simulink model "practica3_PT"  (R2015a)
settings: Solver=ode4  StartTime=0.0  StopTime=1  FixedStep=.005  RelTol=1e-3
settings Model: Creator=Sala6  LastModifiedBy=Jesus

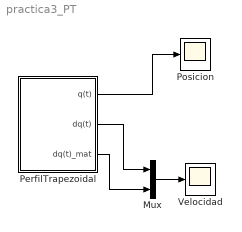
== system practica3_PT ==
  Mux : Mux  Inputs=2
  PerfilTrapezoidal : Subsystem  mask{tf=1, V=60, q0=0, qf=40}
      mask prompts: tf "Tiempo final"; V "Velocidad del perfil"; q0 "Posicion inicial"; qf "Posicion final"
      mask init:
      | % tiempo de mezcla
      | tb=(q0-qf+V*tf)/V
      | a=V/tb
  Posicion : Scope
  Velocidad : Scope
  wires:
  Mux/1 -> Velocidad/1
  PerfilTrapezoidal/2(dq(t)) -> Mux/1
  PerfilTrapezoidal/3(dq(t)_mat) -> Mux/2
  PerfilTrapezoidal/1("q(t) ") -> Posicion/1

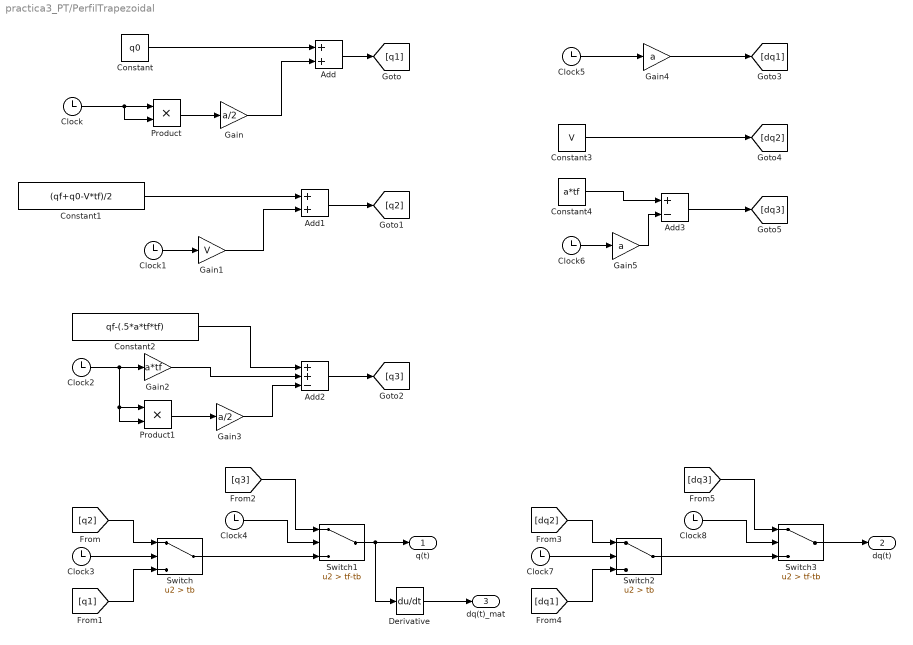
== system practica3_PT/PerfilTrapezoidal ==
  Add : Sum
  Add1 : Sum
  Add2 : Sum  Inputs=++-
  Add3 : Sum  Inputs=+-
  Clock{,1..8} (9 alike) : Clock
  Constant : Constant  Value=q0
  Constant1 : Constant  Value=(qf+q0-V*tf)/2
  Constant2 : Constant  Value=qf-(.5*a*tf*tf)
  Constant3 : Constant  Value=V
  Constant4 : Constant  Value=a*tf
  Derivative : Derivative
  Gain : Gain  Gain=a/2
  Gain1 : Gain  Gain=V
  Gain2 : Gain  Gain=a*tf
  Gain3 : Gain  Gain=a/2
  Gain4 : Gain  Gain=a
  Gain5 : Gain  Gain=a
  Product : Product
  Product1 : Product
  Switch : Switch  Criteria=u2 > Threshold  Threshold=tb
  Switch1 : Switch  Criteria=u2 > Threshold  Threshold=tf-tb
  Switch2 : Switch  Criteria=u2 > Threshold  Threshold=tb
  Switch3 : Switch  Criteria=u2 > Threshold  Threshold=tf-tb
  "q(t) " : Outport
  dq(t) : Outport  Port=2
  dq(t)_mat : Outport  Port=3
  wires:
  Clock3/1 -> Switch/2
  Add/1 -> [q1]
  Switch/1 -> Switch1/3
  [dq1] -> Switch2/3
  [q3] -> Switch1/1
  Constant2/1 -> Add2/1
  Product/1 -> Gain/1
  Clock6/1 -> Gain5/1
  Constant/1 -> Add/1
  Gain/1 -> Add/2
  Product1/1 -> Gain3/1
  Gain3/1 -> Add2/3
  Add1/1 -> [q2]
  Clock8/1 -> Switch3/2
  Clock4/1 -> Switch1/2
  Gain1/1 -> Add1/2
  [dq2] -> Switch2/1
  Switch3/1 -> dq(t)/1
  Add2/1 -> [q3]
  Clock2/1 -> Gain2/1, Product1/1, Product1/2
  Gain5/1 -> Add3/2
  Constant1/1 -> Add1/1
  Clock/1 -> Product/2, Product/1
  Gain2/1 -> Add2/2
  [dq3] -> Switch3/1
  Switch2/1 -> Switch3/3
  Add3/1 -> [dq3]
  Clock7/1 -> Switch2/2
  Clock1/1 -> Gain1/1
  [q2] -> Switch/1
  [q1] -> Switch/3
  Switch1/1 -> "q(t) "/1, Derivative/1
  Constant4/1 -> Add3/1
  Constant3/1 -> [dq2]
  Clock5/1 -> Gain4/1
  Gain4/1 -> [dq1]
  Derivative/1 -> dq(t)_mat/1
